simulink model "ModeloSK"  (R2023a)
settings: Solver=FixedStepAuto  StartTime=0.0  StopTime=Tsim  FixedStep=Ts  RelTol=1e-3
undefined symbols (not defined in the file): K, Kc, t0, Tau, Ti, X0
libraries: fuzblock x1
settings Model: Creator=auditorio  LastModifiedBy=willi
settings OptimizationCC: ReuseModelBlockBuffer=off

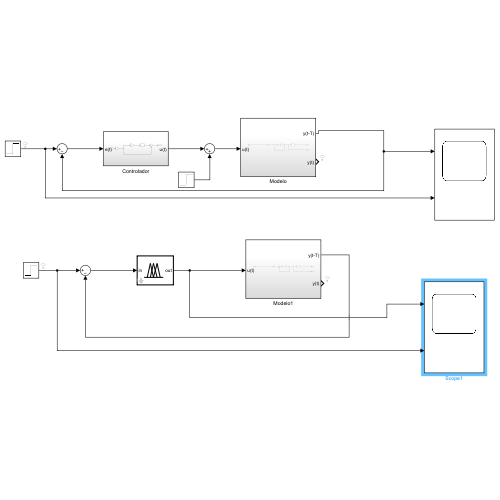
[thumbnail: Simulink's stored preview of the top-level diagram]
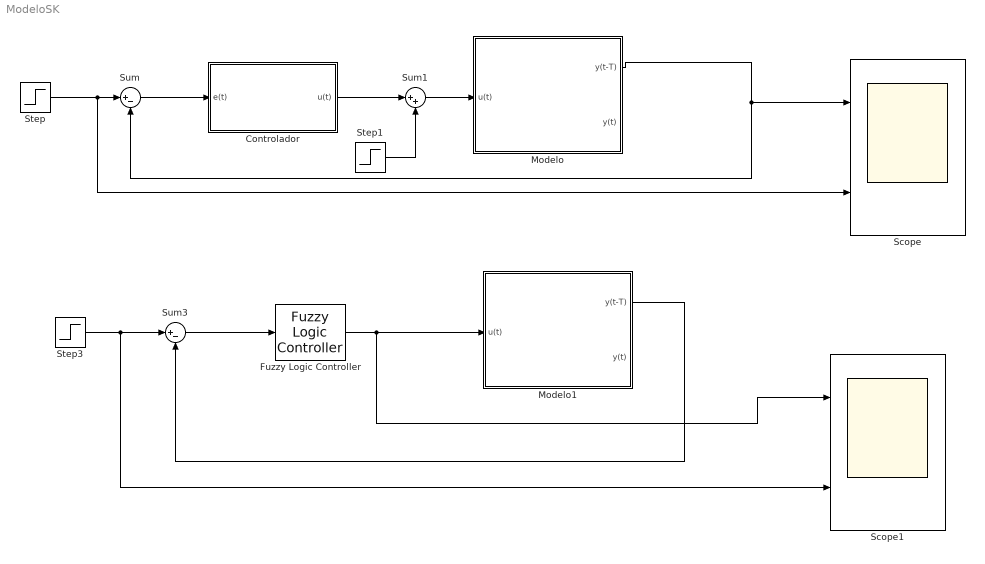
== system ModeloSK ==
  Controlador : Subsystem
  Fuzzy Logic Controller : fuzblock/Fuzzy Logic  Controller  FIS=Fuzzy  OutputSampleNumber=101  DataType=double  FuzzifiedInputs=off  RuleFiringStrengths=off  RuleOutputs=off  AggregatedOutputs=off  SimulateUsing=Interpreted execution  OutOfRangeInputValueMessage=warning  NoRuleFiredMessage=warning  EmptyOutputFuzzySetMessage=warning
  Modelo : Subsystem
  Modelo1 : Subsystem
  Scope : Scope  NumInputPorts=2
  Scope1 : Scope  NumInputPorts=2
  Step : Step  Time=250  Before=X0  After=0.3  SampleTime=0
  Step1 : Step  Time=500  After=0.01  SampleTime=0
  Step3 : Step  Time=250  Before=X0  After=0.3  SampleTime=0
  Sum : Sum  Inputs=|+-
  Sum1 : Sum  Inputs=|++
  Sum3 : Sum  Inputs=|+-
  wires:
  Modelo/1(y(t-T)) -> Sum/2, Scope/1
  Sum/1 -> Controlador/1(e(t))
  Step/1 -> Scope/2, Sum/1
  Controlador/1(u(t)) -> Sum1/1
  Sum1/1 -> Modelo/1(u(t))
  Step1/1 -> Sum1/2
  Sum3/1 -> Fuzzy Logic Controller/1
  Step3/1 -> Scope1/2, Sum3/1
  Modelo1/1(y(t-T)) -> Sum3/2
  Fuzzy Logic Controller/1 -> Scope1/1, Modelo1/1(u(t))

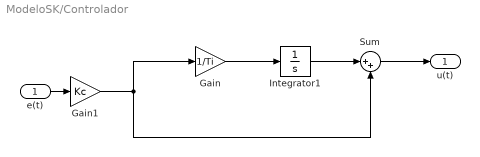
== system ModeloSK/Controlador ==
  e(t) : Inport
  Gain : Gain  Gain=1/Ti
  Gain1 : Gain  Gain=Kc
  Integrator1 : Integrator  InitialCondition=X0/K
  Sum : Sum  Inputs=|++
  u(t) : Outport
  wires:
  Gain1/1 -> Sum/2, Gain/1
  Gain/1 -> Integrator1/1
  Integrator1/1 -> Sum/1
  Sum/1 -> u(t)/1
  e(t)/1 -> Gain1/1

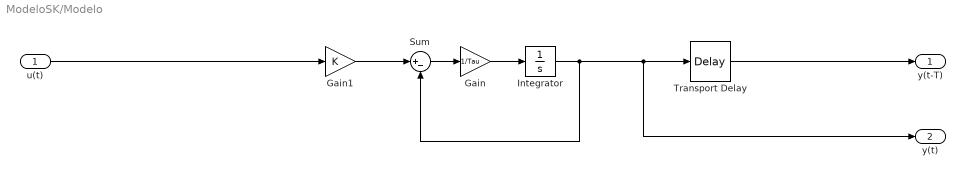
== system ModeloSK/Modelo ==
  u(t) : Inport
  Gain : Gain  Gain=1/Tau
  Gain1 : Gain  Gain=K
  Integrator : Integrator  InitialCondition=X0
  Sum : Sum  Inputs=|+-
  Transport Delay : TransportDelay  DelayTime=t0  InitialOutput=X0
  y(t-T) : Outport
  y(t) : Outport  Port=2
  wires:
  Integrator/1 -> y(t)/1, Transport Delay/1, Sum/2
  Sum/1 -> Gain/1
  Gain/1 -> Integrator/1
  Gain1/1 -> Sum/1
  Transport Delay/1 -> y(t-T)/1
  u(t)/1 -> Gain1/1

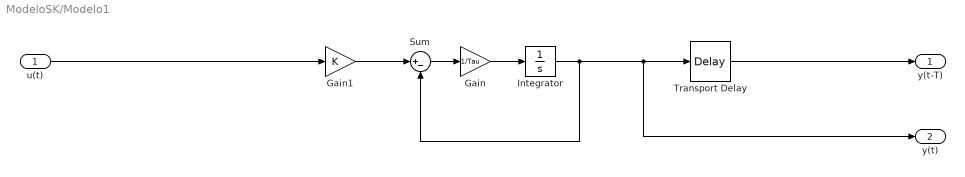
== system ModeloSK/Modelo1 ==
  u(t) : Inport
  Gain : Gain  Gain=1/Tau
  Gain1 : Gain  Gain=K
  Integrator : Integrator  InitialCondition=X0
  Sum : Sum  Inputs=|+-
  Transport Delay : TransportDelay  DelayTime=t0  InitialOutput=X0
  y(t-T) : Outport
  y(t) : Outport  Port=2
  wires:
  Integrator/1 -> y(t)/1, Transport Delay/1, Sum/2
  Sum/1 -> Gain/1
  Gain/1 -> Integrator/1
  Gain1/1 -> Sum/1
  Transport Delay/1 -> y(t-T)/1
  u(t)/1 -> Gain1/1
